simulink model "sst_dab_ttype_inv"  (R2026a)
settings: Solver=ode23tb  StopTime=simlength  FixedStep=tc  MaxStep=glb_time.tc
values from neighbouring files (symbols this model uses):
  afe_ctrl = ctrl_afe_setup(glb_time.ts_afe, grid_emu.omega_grid_nom)    [init_model.m]
  glb_time = timing_setup(fpwm_afe, trgo_afe, fpwm_inv, trgo_inv, fpwm_dab, trgo_dab,                  fpwm_cllc, trgo_cllc, t_measure, tc_factor, tc_decimation, delay_pwm, dead_time_afe,                  dead_time_inv, dead_time_dab, dead_time_cllc)    [init_model.m]
  grid_emu = grid_three_phase_emulator('Dyn11', delta_star, grid_nominal_power, application_voltage, us1, us2, fgrid,                  eq_grid_inductance, eq_grid_resistance, eta, ucc, i1m, p_iron, n1, n2, core_area, core_length, mur,                  up_xi_pu_ref, up_eta_pu_ref, un_xi_pu_ref, un_eta_pu_ref)    [init_model.m]
  omega_set = frequency_set*2*pi    (= 314.159265359)    [init_model.m]
  single_phase_inverter_ctrl = ctrl_single_phase_inverter_setup(glb_time.ts_inv, pres_ctrl.omega_set,      dqvector_pi.kp_inv, dqvector_pi.ki_inv, pres_ctrl.kp_rpi, pres_ctrl.ki_rpi, pres_ctrl.delta_rpi)    [init_model.m]
  sst_num_of_modules = 2    [init_model.m]
undefined symbols (not defined in the file or in its folder): hwdata
libraries: fl_lib x66, nesl_utility x38, pi_ctrl x4, full_bridge_ideal_switch x4, full_bridge_mosfet_based_with_thermal_model x4, full_bridge_mosfet_based_with_thermal_model_zvs x4, discrete_time_low_pass_filter x4, lithium_ion_battery x2, dab_single_phase_pwm_modulator x2, single_phase_transformer x2, dclink_for_three_levels x2, full_bridge_three_level_ttype_ideal_switch_based_model x2
(part 4 of 5)

== system sst_dab_ttype_inv/dab_modA/dcdc_with_galvanic_isolation/full-bridge_2/full-bridge_mosfet_based_with_thermal_model_zvs ==
  gate_commands : Inport
  data_measure : Subsystem
  full-bridge_mosfet_based_ with_thermal_model_zvs : full_bridge_mosfet_based_with_thermal_model_zvs/full-bridge_mosfet_based_ with_thermal_model_zvs  mass_heatsink_m=heatsink.no_weight  specific_heat_m=heatsink.cp  rth_mosfet_HA_m=heatsink.Rth_mosfet_HA  rth_mosfet_JH_m=mosfet.dab.Rth_mosfet_JH  Rds_on_m=mosfet.dab.Rds_on  Vth_m=mosfet.dab.Vth  Eon_m=mosfet.dab.Eon  Eoff_m=mosfet.dab.Eoff  Voff_sw_loss_m=mosfet.dab.Voff_sw_losses  Ion_sw_loss_m=mosfet.dab.Ion_sw_losses  Vdon_diode_m=mosfet.dab.Vdon_diode  Rdon_diode_m=mosfet.dab.Rds_on  JunctionTermalMass_m=mosfet.dab.JunctionTermalMass  Tambient_m=heatsink.Tambient  DThs_init_m=heatsink.DThs_init  Csnubber_m=mosfet.dab.Csnubber_zvs  Rsnubber_m=mosfet.dab.Rsnubber_zvs
  udc(+) : PMIOPort  Side=Left
  udc(-) : PMIOPort  Port=2  Side=Left
  uac(+) : PMIOPort  Port=3  Side=Right
  uac(-) : PMIOPort  Port=4  Side=Right
  wires:
  full-bridge_mosfet_based_ with_thermal_model_zvs/1 -> data_measure/1(m)
  gate_commands/1 -> full-bridge_mosfet_based_ with_thermal_model_zvs/1
  connections:
  full-bridge_mosfet_based_ with_thermal_model_zvs/LConn2 -- udc(-)/RConn1
  full-bridge_mosfet_based_ with_thermal_model_zvs/LConn1 -- udc(+)/RConn1
  full-bridge_mosfet_based_ with_thermal_model_zvs/RConn2 -- uac(-)/RConn1
  full-bridge_mosfet_based_ with_thermal_model_zvs/RConn1 -- uac(+)/RConn1

== system sst_dab_ttype_inv/dab_modB/dab_ctrl/dab_voltage&current_controllers/input current controller ==
  i_in_dab_ref : Inport
  i_in_dab : Inport  Port=2
  Gain : Gain
  dab_current_control performance_modA : Scope  NumInputPorts=3
      settings: ActiveDisplayYMinimum=-1.3198512407012277  ActiveDisplayYMaximum=3.2550260581251234  DataLoggingVariableName=ScopeData12
  pi_ctrl : pi_ctrl/pi_ctrl  kp=dab_ctrl.kp_idc  ki=dab_ctrl.ki_idc  ts=glb_time.ts_dab  lim_up=1  lim_down=-1
  i_ctrl_out : Outport
  wires:
  i_in_dab_ref/1 -> pi_ctrl/1, dab_current_control performance_modA/1, Gain/1  "i_in_dab_ref"
  i_in_dab/1 -> pi_ctrl/2, dab_current_control performance_modA/2  "i_in_dab"
  pi_ctrl/1 -> i_ctrl_out/1, dab_current_control performance_modA/3  "i_ctrl_out"
  Gain/1 -> pi_ctrl/3

== system sst_dab_ttype_inv/dab_modB/dab_ctrl/dab_voltage&current_controllers/output voltage controller ==
  u_out_dab_ref : Inport
  u_out_dab : Inport  Port=2
  dab_voltage_control performance_modA : Scope  NumInputPorts=3
      settings: ActiveDisplayYMinimum=-1.3198512407012277  ActiveDisplayYMaximum=3.2550260581251234  DataLoggingVariableName=ScopeData14
  pi_ctrl : pi_ctrl/pi_ctrl  kp=dab_ctrl.kp_udc  ki=dab_ctrl.ki_udc  ts=glb_time.ts_dab  lim_up=1  lim_down=-1
  u_ctrl_out : Outport
  wires:
  u_out_dab/1 -> dab_voltage_control performance_modA/2, pi_ctrl/2  "u_out_dab"
  u_out_dab_ref/1 -> dab_voltage_control performance_modA/1, pi_ctrl/3, pi_ctrl/1  "u_out_dab_ref"
  pi_ctrl/1 -> dab_voltage_control performance_modA/3, u_ctrl_out/1  "u_ctrl_out"

== system sst_dab_ttype_inv/dab_modB/dab_ctrl/dab_voltage&current_controllers/scopes ==
  Bus Creator : BusCreator  Inputs=2
  Bus Creator1 : BusCreator  Inputs=2
  dab-tracking modA : Scope  NumInputPorts=2
      settings: ActiveDisplayYMinimum=-2.2033655574404327  ActiveDisplayYMaximum=2.9011172646804795  DataLoggingVariableName=ScopeData7
  u_ctrl_out_dab/i_ctrl_out_dab modA : Scope  NumInputPorts=2
      settings: ActiveDisplayYMinimum=-1.25  ActiveDisplayYMaximum=1.25
  wires:
  [dab_current_input_pu] -> Bus Creator1/2  "dab_current_input_pu"
  [dab_current_ctrl_output_pu] -> u_ctrl_out_dab/i_ctrl_out_dab modA/2  "i_ctrl_out_dab"
  [dab_voltage_output_pu] -> Bus Creator/2  "dab_voltage_output_pu"
  [dab_voltage_output_pu_reference] -> Bus Creator/1  "dab_current_input_pu_ref"
  Bus Creator1/1 -> dab-tracking modA/2
  Bus Creator/1 -> dab-tracking modA/1
  [dab_voltage_ctrl_output_pu] -> u_ctrl_out_dab/i_ctrl_out_dab modA/1  "u_ctrl_out_dab"
  [dab_voltage_ctrl_output_pu] -> Bus Creator1/1  "u_ctrl_out_dab"

== system sst_dab_ttype_inv/dab_modB/dab_ctrl/dab_voltage&current_controllers/storage_data_dab ==
  To Workspace1 : ToWorkspace  VariableName=time_ts_dab_sim  SampleTime=-1
      settings: MaxDataPoints=Ns_dab
  To Workspace2 : ToWorkspace  VariableName=dab_current_input_pu_ref_sim  SampleTime=-1
      settings: MaxDataPoints=Ns_dab
  To Workspace3 : ToWorkspace  VariableName=dab_voltage_output_pu_sim  SampleTime=-1
      settings: MaxDataPoints=Ns_dab
  To Workspace5 : ToWorkspace  VariableName=dab_current_input_pu_sim  SampleTime=-1
      settings: MaxDataPoints=Ns_dab
  To Workspace6 : ToWorkspace  VariableName=u_ctrl_out_dab_sim  SampleTime=-1
      settings: MaxDataPoints=Ns_dab
  To Workspace7 : ToWorkspace  VariableName=i_ctrl_out_dab_sim  SampleTime=-1
      settings: MaxDataPoints=Ns_dab
  wires:
  [dab_voltage_ctrl_output_pu] -> To Workspace6/1  "u_ctrl_out_dab"
  [dab_voltage_output_pu_reference] -> To Workspace2/1  "dab_current_input_pu_ref"
  [dab_voltage_output_pu] -> To Workspace3/1  "dab_voltage_output_pu"
  [dab_current_ctrl_output_pu] -> To Workspace7/1  "i_ctrl_out_dab"
  [dab_current_input_pu] -> To Workspace5/1  "dab_current_input_pu"
  [time_dab_module_2] -> To Workspace1/1

== system sst_dab_ttype_inv/dab_modB/dcdc_with_galvanic_isolation/full-bridge_1/full-bridge_ideal_switch_based ==
  gate_commands : Inport
  data_measure : Subsystem
  full-bridge_ideal_switch_based : full_bridge_ideal_switch/full-bridge ideal switch based  Rds_on=ideal_switch.dab.Rds_on  Vdon_diode=ideal_switch.dab.Vdon_diode  Rdon_diode=ideal_switch.dab.Rdon_diode  Csnubber=ideal_switch.dab.Csnubber_zvs  Rsnubber=ideal_switch.dab.Rsnubber_zvs  Vth=ideal_switch.dab.Vth
  udc(+) : PMIOPort  Side=Left
  uac(+) : PMIOPort  Port=2  Side=Right
  udc(-) : PMIOPort  Port=3  Side=Left
  uac(-) : PMIOPort  Port=4  Side=Right
  wires:
  gate_commands/1 -> full-bridge_ideal_switch_based/1
  full-bridge_ideal_switch_based/1 -> data_measure/1(m)
  connections:
  uac(-)/RConn1 -- full-bridge_ideal_switch_based/RConn2
  full-bridge_ideal_switch_based/RConn1 -- uac(+)/RConn1
  udc(-)/RConn1 -- full-bridge_ideal_switch_based/LConn2
  udc(+)/RConn1 -- full-bridge_ideal_switch_based/LConn1

== system sst_dab_ttype_inv/dab_modB/dcdc_with_galvanic_isolation/full-bridge_1/full-bridge_mosfet_based_with_thermal_model ==
  gate_commands : Inport
  data_measure : Subsystem
  full-bridge_mosfet_based_with_thermal_model : full_bridge_mosfet_based_with_thermal_model/full-bridge mosfet based with thermal model  mass_heatsink_m=heatsink.no_weight  specific_heat_m=heatsink.cp  rth_mosfet_HA_m=heatsink.Rth_mosfet_HA  rth_mosfet_JH_m=mosfet.dab.Rth_mosfet_JH  Rds_on_m=mosfet.dab.Rds_on  Vth_m=mosfet.dab.Vth  Eon_m=mosfet.dab.Eon  Eoff_m=mosfet.dab.Eoff  Voff_sw_loss_m=mosfet.dab.Voff_sw_losses  Ion_sw_loss_m=mosfet.dab.Ion_sw_losses  Vdon_diode_m=mosfet.dab.Vdon_diode  Rdon_diode_m=mosfet.dab.Rds_on  JunctionTermalMass_m=mosfet.dab.JunctionTermalMass  Tambient_m=heatsink.Tambient  DThs_init_m=heatsink.DThs_init
  udc(+) : PMIOPort  Side=Left
  uac(+) : PMIOPort  Port=2  Side=Right
  udc(-) : PMIOPort  Port=3  Side=Left
  uac(-) : PMIOPort  Port=4  Side=Right
  wires:
  gate_commands/1 -> full-bridge_mosfet_based_with_thermal_model/1
  full-bridge_mosfet_based_with_thermal_model/1 -> data_measure/1(m)
  connections:
  full-bridge_mosfet_based_with_thermal_model/RConn1 -- uac(+)/RConn1
  udc(-)/RConn1 -- full-bridge_mosfet_based_with_thermal_model/LConn2
  full-bridge_mosfet_based_with_thermal_model/LConn1 -- udc(+)/RConn1
  full-bridge_mosfet_based_with_thermal_model/RConn2 -- uac(-)/RConn1

== system sst_dab_ttype_inv/dab_modB/dcdc_with_galvanic_isolation/full-bridge_1/full-bridge_mosfet_based_with_thermal_model_zvs ==
  gate_commands : Inport
  data_measure : Subsystem
  full-bridge_mosfet_based_ with_thermal_model_zvs : full_bridge_mosfet_based_with_thermal_model_zvs/full-bridge_mosfet_based_ with_thermal_model_zvs  mass_heatsink_m=heatsink.no_weight  specific_heat_m=heatsink.cp  rth_mosfet_HA_m=heatsink.Rth_mosfet_HA  rth_mosfet_JH_m=mosfet.dab.Rth_mosfet_JH  Rds_on_m=mosfet.dab.Rds_on  Vth_m=mosfet.dab.Vth  Eon_m=mosfet.dab.Eon  Eoff_m=mosfet.dab.Eoff  Voff_sw_loss_m=mosfet.dab.Voff_sw_losses  Ion_sw_loss_m=mosfet.dab.Ion_sw_losses  Vdon_diode_m=mosfet.dab.Vdon_diode  Rdon_diode_m=mosfet.dab.Rds_on  JunctionTermalMass_m=mosfet.dab.JunctionTermalMass  Tambient_m=heatsink.Tambient  DThs_init_m=heatsink.DThs_init  Csnubber_m=mosfet.dab.Csnubber_zvs  Rsnubber_m=mosfet.dab.Rsnubber_zvs
  udc(+) : PMIOPort  Side=Left
  udc(-) : PMIOPort  Port=2  Side=Left
  uac(+) : PMIOPort  Port=3  Side=Right
  uac(-) : PMIOPort  Port=4  Side=Right
  wires:
  gate_commands/1 -> full-bridge_mosfet_based_ with_thermal_model_zvs/1
  full-bridge_mosfet_based_ with_thermal_model_zvs/1 -> data_measure/1(m)
  connections:
  full-bridge_mosfet_based_ with_thermal_model_zvs/RConn1 -- uac(+)/RConn1
  full-bridge_mosfet_based_ with_thermal_model_zvs/RConn2 -- uac(-)/RConn1
  full-bridge_mosfet_based_ with_thermal_model_zvs/LConn1 -- udc(+)/RConn1
  full-bridge_mosfet_based_ with_thermal_model_zvs/LConn2 -- udc(-)/RConn1

== system sst_dab_ttype_inv/dab_modB/dcdc_with_galvanic_isolation/full-bridge_2/full-bridge_ideal_switch_based ==
  gate_commands : Inport
  data_measure : Subsystem
  full-bridge_ideal_switch_based : full_bridge_ideal_switch/full-bridge ideal switch based  Rds_on=ideal_switch.dab.Rds_on  Vdon_diode=ideal_switch.dab.Vdon_diode  Rdon_diode=ideal_switch.dab.Rdon_diode  Csnubber=ideal_switch.dab.Csnubber_zvs  Rsnubber=ideal_switch.dab.Rsnubber_zvs  Vth=ideal_switch.dab.Vth
  udc(+) : PMIOPort  Side=Left
  uac(+) : PMIOPort  Port=2  Side=Right
  udc(-) : PMIOPort  Port=3  Side=Left
  uac(-) : PMIOPort  Port=4  Side=Right
  wires:
  gate_commands/1 -> full-bridge_ideal_switch_based/1
  full-bridge_ideal_switch_based/1 -> data_measure/1(m)
  connections:
  uac(-)/RConn1 -- full-bridge_ideal_switch_based/RConn2
  full-bridge_ideal_switch_based/RConn1 -- uac(+)/RConn1
  udc(-)/RConn1 -- full-bridge_ideal_switch_based/LConn2
  udc(+)/RConn1 -- full-bridge_ideal_switch_based/LConn1

== system sst_dab_ttype_inv/dab_modB/dcdc_with_galvanic_isolation/full-bridge_2/full-bridge_mosfet_based_with_thermal_model ==
  gate_commands : Inport
  data_measure : Subsystem
  full-bridge_mosfet_based_with_thermal_model : full_bridge_mosfet_based_with_thermal_model/full-bridge mosfet based with thermal model  mass_heatsink_m=heatsink.no_weight  specific_heat_m=heatsink.cp  rth_mosfet_HA_m=heatsink.Rth_mosfet_HA  rth_mosfet_JH_m=mosfet.dab.Rth_mosfet_JH  Rds_on_m=mosfet.dab.Rds_on  Vth_m=mosfet.dab.Vth  Eon_m=mosfet.dab.Eon  Eoff_m=mosfet.dab.Eoff  Voff_sw_loss_m=mosfet.dab.Voff_sw_losses  Ion_sw_loss_m=mosfet.dab.Ion_sw_losses  Vdon_diode_m=mosfet.dab.Vdon_diode  Rdon_diode_m=mosfet.dab.Rds_on  JunctionTermalMass_m=mosfet.dab.JunctionTermalMass  Tambient_m=heatsink.Tambient  DThs_init_m=heatsink.DThs_init
  udc(+) : PMIOPort  Side=Left
  uac(+) : PMIOPort  Port=2  Side=Right
  udc(-) : PMIOPort  Port=3  Side=Left
  uac(-) : PMIOPort  Port=4  Side=Right
  wires:
  gate_commands/1 -> full-bridge_mosfet_based_with_thermal_model/1
  full-bridge_mosfet_based_with_thermal_model/1 -> data_measure/1(m)
  connections:
  full-bridge_mosfet_based_with_thermal_model/RConn1 -- uac(+)/RConn1
  udc(-)/RConn1 -- full-bridge_mosfet_based_with_thermal_model/LConn2
  full-bridge_mosfet_based_with_thermal_model/LConn1 -- udc(+)/RConn1
  full-bridge_mosfet_based_with_thermal_model/RConn2 -- uac(-)/RConn1

== system sst_dab_ttype_inv/dab_modB/dcdc_with_galvanic_isolation/full-bridge_2/full-bridge_mosfet_based_with_thermal_model_zvs ==
  gate_commands : Inport
  data_measure : Subsystem
  full-bridge_mosfet_based_ with_thermal_model_zvs : full_bridge_mosfet_based_with_thermal_model_zvs/full-bridge_mosfet_based_ with_thermal_model_zvs  mass_heatsink_m=heatsink.no_weight  specific_heat_m=heatsink.cp  rth_mosfet_HA_m=heatsink.Rth_mosfet_HA  rth_mosfet_JH_m=mosfet.dab.Rth_mosfet_JH  Rds_on_m=mosfet.dab.Rds_on  Vth_m=mosfet.dab.Vth  Eon_m=mosfet.dab.Eon  Eoff_m=mosfet.dab.Eoff  Voff_sw_loss_m=mosfet.dab.Voff_sw_losses  Ion_sw_loss_m=mosfet.dab.Ion_sw_losses  Vdon_diode_m=mosfet.dab.Vdon_diode  Rdon_diode_m=mosfet.dab.Rds_on  JunctionTermalMass_m=mosfet.dab.JunctionTermalMass  Tambient_m=heatsink.Tambient  DThs_init_m=heatsink.DThs_init  Csnubber_m=mosfet.dab.Csnubber_zvs  Rsnubber_m=mosfet.dab.Rsnubber_zvs
  udc(+) : PMIOPort  Side=Left
  udc(-) : PMIOPort  Port=2  Side=Left
  uac(+) : PMIOPort  Port=3  Side=Right
  uac(-) : PMIOPort  Port=4  Side=Right
  wires:
  gate_commands/1 -> full-bridge_mosfet_based_ with_thermal_model_zvs/1
  full-bridge_mosfet_based_ with_thermal_model_zvs/1 -> data_measure/1(m)
  connections:
  full-bridge_mosfet_based_ with_thermal_model_zvs/RConn1 -- uac(+)/RConn1
  full-bridge_mosfet_based_ with_thermal_model_zvs/RConn2 -- uac(-)/RConn1
  full-bridge_mosfet_based_ with_thermal_model_zvs/LConn1 -- udc(+)/RConn1
  full-bridge_mosfet_based_ with_thermal_model_zvs/LConn2 -- udc(-)/RConn1

== system sst_dab_ttype_inv/single_phase_inverter_modA/single phase inverter control/single_phase_inverter_ctrl/scopes ==
  Bus Creator1 : BusCreator  Inputs=3
  Bus Creator2 : BusCreator  Inputs=2
  Bus Creator3 : BusCreator  Inputs=2
  Bus Creator4 : BusCreator  Inputs=2
  single phase inverter tracking current scope 1 : Scope  NumInputPorts=2
      settings: ActiveDisplayYMinimum=-1.23468017578125  ActiveDisplayYMaximum=1.23419189453125  DataLoggingVariableName=ScopeData12
  single phase inverter tracking current scope 2 : Scope  NumInputPorts=2
      settings: ActiveDisplayYMinimum=-3.07452392578125  ActiveDisplayYMaximum=2.19708251953125  DataLoggingVariableName=ScopeData2
  wires:
  Bus Creator1/1 -> single phase inverter tracking current scope 1/2  "is_tracking"
  [i_out_alphabeta_ref] -> Bus Creator1/2  "i_out_inverter_pu_ref"
  [afe_current_output_pu] -> Bus Creator1/3  "inverter_current_output_pu"
  [afe_voltage_output_pu] -> Bus Creator2/1  "inverter_voltage_output_pu"
  Bus Creator2/1 -> single phase inverter tracking current scope 1/1  "load"
  [inverter_current_output_pu_reference] -> Bus Creator1/1  "inverter_current_output_pu_reference"
  [afe_current_output_pu] -> Bus Creator2/2  "inverter_current_output_pu"
  [u_ctrl_out] -> Bus Creator3/1  "u_ctrl_out"
  [afe_voltage_output_pu] -> Bus Creator3/2  "inverter_voltage_output_pu"
  Bus Creator3/1 -> single phase inverter tracking current scope 2/2  "u_load"
  [afe_current_output_pu] -> Bus Creator4/2  "inverter_current_output_pu"
  [i_out_alphabeta_ref] -> Bus Creator4/1  "i_out_alphabeta_ref"
  Bus Creator4/1 -> single phase inverter tracking current scope 2/1  "i_load"

== system sst_dab_ttype_inv/single_phase_inverter_modA/single phase inverter control/single_phase_inverter_ctrl/single_phase_current_control ==
  inverter_current_output_pu_reference : Inport
  current_reference_generation : Subsystem
  dqpi_current_controller : Subsystem
  u_ctrl_out : Outport
  tag scope: i_out_alphabeta_ref=scoped, inverter_current_output_pu_reference=scoped, u_ctrl_out=scoped
  wires:
  current_reference_generation/1(is_ref) -> [i_out_alphabeta_ref]  "i_out_inverter_pu_ref"
  dqpi_current_controller/1(u_out) -> u_ctrl_out/1, [u_ctrl_out]  "u_ctrl_out"
  [phase_grid] -> current_reference_generation/2(phase)
  inverter_current_output_pu_reference/1 -> current_reference_generation/1(mag_ref), [inverter_current_output_pu_reference]
  current_reference_generation/2(id_ref) -> dqpi_current_controller/1(id_ref)

== system sst_dab_ttype_inv/single_phase_inverter_modA/single phase inverter control/single_phase_inverter_ctrl/single_phase_pll ==
  input : Inport
  Constant : Constant
  Constant2 : Constant  Value=0
  Scope : Scope  NumInputPorts=2
      settings: ActiveDisplayYMinimum=-3.2854912154015015  ActiveDisplayYMaximum=3.4773424919151528
  Sum : Sum  Inputs=|++
  Sum1 : Sum  Inputs=|++
  Terminator : Terminator
  Terminator1 : Terminator
  Terminator2 : Terminator
  Unit Delay1 : UnitDelay  SampleTime=-1
  alphabeta2xieta : MATLAB Function  TreatAsAtomicUnit=on
  bounder2 : MATLAB Function  TreatAsAtomicUnit=on
  double_integrator_observer : Subsystem
  freq_pll : Gain  Gain=1/2/pi
  omega_int_ts : Gain  Gain=omega_set * glb_time.ts_inv
  pi-ctrl : Subsystem  mask{kp=1, ki=0, ts=glb_time.ts_inv, sat_pos=2, sat_neg=-2}
  ualpha_pll : Gain
  ubeta_pll : Gain
  ueta_pll : Gain  Gain=-1
  ueta_pll_flt : discrete_time_low_pass_filter/discrete-time-low-pass-filter  tau=2/omega_set  ts=glb_time.ts_inv
  uxi_pll : Gain
  uxi_pll_flt : discrete_time_low_pass_filter/discrete-time-low-pass-filter  tau=2/omega_set  ts=glb_time.ts_inv
  xieta2alphabeta : MATLAB Function  TreatAsAtomicUnit=on
  phase_pll_hat : Outport
  omega_pll_hat : Outport  Port=2
  wires:
  Sum/1 -> bounder2/1(u)
  alphabeta2xieta/1(xi) -> uxi_pll/1, uxi_pll_flt/1
  xieta2alphabeta/2(beta) -> ubeta_pll/1
  alphabeta2xieta/2(eta) -> ueta_pll/1, ueta_pll_flt/1
  omega_int_ts/1 -> freq_pll/1, Sum/1
  double_integrator_observer/1(phase_hat) -> Scope/1, phase_pll_hat/1  "phase_pll_hat"
  input/1 -> alphabeta2xieta/1(alpha)
  freq_pll/1 -> Terminator1/1  "freq_pll"
  ueta_pll_flt/1 -> xieta2alphabeta/2(eta)
  uxi_pll_flt/1 -> xieta2alphabeta/1(xi)
  ueta_pll/1 -> pi-ctrl/1(x)
  Sum1/1 -> omega_int_ts/1  "freq_pll"
  Constant2/1 -> pi-ctrl/2(xref)
  uxi_pll/1 -> Terminator2/1
  ubeta_pll/1 -> alphabeta2xieta/2(beta)
  xieta2alphabeta/1(alpha) -> ualpha_pll/1
  pi-ctrl/1(u) -> Sum1/1
  Constant/1 -> Sum1/2
  Unit Delay1/1 -> Sum/2, alphabeta2xieta/3(gamma), xieta2alphabeta/3(gamma), double_integrator_observer/1(theta)
  bounder2/1(y) -> Unit Delay1/1  "theta_hat_bounded"
  double_integrator_observer/2(omega_hat) -> Scope/2, omega_pll_hat/1  "omega_pll_hat"
  ualpha_pll/1 -> Terminator/1

== system sst_dab_ttype_inv/single_phase_inverter_modA/single phase inverter control/single_phase_inverter_ctrl/storage_data ==
  To Workspace : ToWorkspace  VariableName=inverter_voltage_output_pu_sim  SampleTime=-1
      settings: MaxDataPoints=glb_time.Ns_inv  Save2DSignal=2-D array (concatenate along first dimension)
  To Workspace1 : ToWorkspace  VariableName=inverter_current_output_pu_sim  SampleTime=-1
      settings: MaxDataPoints=glb_time.Ns_inv  Save2DSignal=2-D array (concatenate along first dimension)
  To Workspace10 : ToWorkspace  VariableName=iq_pu_ref_sim  SampleTime=-1
      settings: MaxDataPoints=glb_time.Ns_inv  Save2DSignal=2-D array (concatenate along first dimension)
  To Workspace11 : ToWorkspace  VariableName=iq_pu_sim  SampleTime=-1
      settings: MaxDataPoints=glb_time.Ns_inv  Save2DSignal=2-D array (concatenate along first dimension)
  To Workspace12 : ToWorkspace  VariableName=ud_ctrl_out_sim  SampleTime=-1
      settings: MaxDataPoints=glb_time.Ns_inv  Save2DSignal=2-D array (concatenate along first dimension)
  To Workspace13 : ToWorkspace  VariableName=uq_ctrl_out_sim  SampleTime=-1
      settings: MaxDataPoints=glb_time.Ns_inv  Save2DSignal=2-D array (concatenate along first dimension)
  To Workspace2 : ToWorkspace  VariableName=inverter_current_output_pu_reference_sim  SampleTime=-1
      settings: MaxDataPoints=glb_time.Ns_inv  Save2DSignal=2-D array (concatenate along first dimension)
  To Workspace3 : ToWorkspace  VariableName=i_out_inverter_pu_ref_sim  SampleTime=-1
      settings: MaxDataPoints=glb_time.Ns_inv  Save2DSignal=2-D array (concatenate along first dimension)
  To Workspace4 : ToWorkspace  VariableName=u_ctrl_out_sim  SampleTime=-1
      settings: MaxDataPoints=glb_time.Ns_inv  Save2DSignal=2-D array (concatenate along first dimension)
  To Workspace5 : ToWorkspace  VariableName=time_ts_inv_sim  SampleTime=-1
      settings: MaxDataPoints=glb_time.Ns_inv  Save2DSignal=2-D array (concatenate along first dimension)
  To Workspace6 : ToWorkspace  VariableName=i_alpha_pu_sim  SampleTime=-1
      settings: MaxDataPoints=glb_time.Ns_inv  Save2DSignal=2-D array (concatenate along first dimension)
  To Workspace7 : ToWorkspace  VariableName=i_beta_pu_sim  SampleTime=-1
      settings: MaxDataPoints=glb_time.Ns_inv  Save2DSignal=2-D array (concatenate along first dimension)
  To Workspace8 : ToWorkspace  VariableName=id_pu_ref_sim  SampleTime=-1
      settings: MaxDataPoints=glb_time.Ns_inv  Save2DSignal=2-D array (concatenate along first dimension)
  To Workspace9 : ToWorkspace  VariableName=id_pu_sim  SampleTime=-1
      settings: MaxDataPoints=glb_time.Ns_inv  Save2DSignal=2-D array (concatenate along first dimension)
  wires:
  [afe_voltage_output_pu] -> To Workspace/1  "inverter_voltage_output_pu"
  [afe_current_output_pu] -> To Workspace1/1  "inverter_current_output_pu"
  [inverter_current_output_pu_reference] -> To Workspace2/1  "inverter_current_output_pu_reference"
  [i_out_alphabeta_ref] -> To Workspace3/1  "i_out_inverter_pu_ref"
  [u_ctrl_out] -> To Workspace4/1  "u_ctrl_out"
  [local_time] -> To Workspace5/1
  [i_alpha] -> To Workspace6/1
  [i_beta] -> To Workspace7/1
  [id_ref] -> To Workspace8/1
  [id] -> To Workspace9/1
  [iq_ref] -> To Workspace10/1
  [iq] -> To Workspace11/1
  [ud_ctrl] -> To Workspace12/1
  [uq_ctrl] -> To Workspace13/1

== system sst_dab_ttype_inv/single_phase_inverter_modB/single phase inverter control/single_phase_inverter_ctrl/scopes ==
  Bus Creator1 : BusCreator  Inputs=3
  Bus Creator2 : BusCreator  Inputs=2
  Bus Creator3 : BusCreator  Inputs=2
  Bus Creator4 : BusCreator  Inputs=2
  single phase inverter tracking current scope 1 : Scope  NumInputPorts=2
      settings: ActiveDisplayYMinimum=-1.23468017578125  ActiveDisplayYMaximum=1.23419189453125  DataLoggingVariableName=ScopeData12
  single phase inverter tracking current scope 2 : Scope  NumInputPorts=2
      settings: ActiveDisplayYMinimum=-1.2603759765625  ActiveDisplayYMaximum=1.2652587890625  DataLoggingVariableName=ScopeData2
  wires:
  Bus Creator4/1 -> single phase inverter tracking current scope 2/1  "i_load"
  [i_out_alphabeta_ref] -> Bus Creator4/1  "i_out_alphabeta_ref"
  [afe_current_output_pu] -> Bus Creator4/2  "inverter_current_output_pu"
  Bus Creator3/1 -> single phase inverter tracking current scope 2/2  "u_load"
  [afe_voltage_output_pu] -> Bus Creator3/2  "inverter_voltage_output_pu"
  [u_ctrl_out] -> Bus Creator3/1  "u_ctrl_out"
  [afe_current_output_pu] -> Bus Creator2/2  "inverter_current_output_pu"
  [inverter_current_output_pu_reference] -> Bus Creator1/1  "inverter_current_output_pu_reference"
  Bus Creator2/1 -> single phase inverter tracking current scope 1/1  "load"
  [afe_voltage_output_pu] -> Bus Creator2/1  "inverter_voltage_output_pu"
  [afe_current_output_pu] -> Bus Creator1/3  "inverter_current_output_pu"
  [i_out_alphabeta_ref] -> Bus Creator1/2  "i_out_inverter_pu_ref"
  Bus Creator1/1 -> single phase inverter tracking current scope 1/2  "is_tracking"

== system sst_dab_ttype_inv/single_phase_inverter_modB/single phase inverter control/single_phase_inverter_ctrl/single_phase_current_control ==
  inverter_current_output_pu_reference : Inport
  current_reference_generation : Subsystem
  dqpi_current_controller : Subsystem
  u_ctrl_out : Outport
  tag scope: i_out_alphabeta_ref=scoped, inverter_current_output_pu_reference=scoped, u_ctrl_out=scoped
  wires:
  current_reference_generation/2(id_ref) -> dqpi_current_controller/1(id_ref)
  inverter_current_output_pu_reference/1 -> [inverter_current_output_pu_reference], current_reference_generation/1(mag_ref)
  [phase_grid] -> current_reference_generation/2(phase)
  dqpi_current_controller/1(u_out) -> [u_ctrl_out], u_ctrl_out/1  "u_ctrl_out"
  current_reference_generation/1(is_ref) -> [i_out_alphabeta_ref]  "i_out_inverter_pu_ref"

== system sst_dab_ttype_inv/single_phase_inverter_modB/single phase inverter control/single_phase_inverter_ctrl/single_phase_pll ==
  input : Inport
  Constant : Constant
  Constant2 : Constant  Value=0
  Scope : Scope  NumInputPorts=2
      settings: ActiveDisplayYMinimum=-3.2854912154015015  ActiveDisplayYMaximum=3.4773424919151528
  Sum : Sum  Inputs=|++
  Sum1 : Sum  Inputs=|++
  Terminator : Terminator
  Terminator1 : Terminator
  Terminator2 : Terminator
  Unit Delay1 : UnitDelay  SampleTime=-1
  alphabeta2xieta : MATLAB Function  TreatAsAtomicUnit=on
  bounder2 : MATLAB Function  TreatAsAtomicUnit=on
  double_integrator_observer : Subsystem
  freq_pll : Gain  Gain=1/2/pi
  omega_int_ts : Gain  Gain=omega_set * glb_time.ts_inv
  pi-ctrl : Subsystem  mask{kp=1, ki=0, ts=glb_time.ts_inv, sat_pos=2, sat_neg=-2}
  ualpha_pll : Gain
  ubeta_pll : Gain
  ueta_pll : Gain  Gain=-1
  ueta_pll_flt : discrete_time_low_pass_filter/discrete-time-low-pass-filter  tau=2/omega_set  ts=glb_time.ts_inv
  uxi_pll : Gain
  uxi_pll_flt : discrete_time_low_pass_filter/discrete-time-low-pass-filter  tau=2/omega_set  ts=glb_time.ts_inv
  xieta2alphabeta : MATLAB Function  TreatAsAtomicUnit=on
  phase_pll_hat : Outport
  omega_pll_hat : Outport  Port=2
  wires:
  ualpha_pll/1 -> Terminator/1
  double_integrator_observer/2(omega_hat) -> omega_pll_hat/1, Scope/2  "omega_pll_hat"
  bounder2/1(y) -> Unit Delay1/1  "theta_hat_bounded"
  Unit Delay1/1 -> double_integrator_observer/1(theta), xieta2alphabeta/3(gamma), alphabeta2xieta/3(gamma), Sum/2
  Constant/1 -> Sum1/2
  pi-ctrl/1(u) -> Sum1/1
  xieta2alphabeta/1(alpha) -> ualpha_pll/1
  ubeta_pll/1 -> alphabeta2xieta/2(beta)
  uxi_pll/1 -> Terminator2/1
  Constant2/1 -> pi-ctrl/2(xref)
  Sum1/1 -> omega_int_ts/1  "freq_pll"
  ueta_pll/1 -> pi-ctrl/1(x)
  uxi_pll_flt/1 -> xieta2alphabeta/1(xi)
  ueta_pll_flt/1 -> xieta2alphabeta/2(eta)
  freq_pll/1 -> Terminator1/1  "freq_pll"
  input/1 -> alphabeta2xieta/1(alpha)
  double_integrator_observer/1(phase_hat) -> phase_pll_hat/1, Scope/1  "phase_pll_hat"
  omega_int_ts/1 -> Sum/1, freq_pll/1
  alphabeta2xieta/2(eta) -> ueta_pll_flt/1, ueta_pll/1
  xieta2alphabeta/2(beta) -> ubeta_pll/1
  alphabeta2xieta/1(xi) -> uxi_pll_flt/1, uxi_pll/1
  Sum/1 -> bounder2/1(u)

== system sst_dab_ttype_inv/single_phase_inverter_modB/single phase inverter control/single_phase_inverter_ctrl/storage_data ==
  To Workspace : ToWorkspace  VariableName=inverter_voltage_output_pu_sim  SampleTime=-1
      settings: MaxDataPoints=glb_time.Ns_inv  Save2DSignal=2-D array (concatenate along first dimension)
  To Workspace1 : ToWorkspace  VariableName=inverter_current_output_pu_sim  SampleTime=-1
      settings: MaxDataPoints=glb_time.Ns_inv  Save2DSignal=2-D array (concatenate along first dimension)
  To Workspace10 : ToWorkspace  VariableName=iq_pu_ref_sim  SampleTime=-1
      settings: MaxDataPoints=glb_time.Ns_inv  Save2DSignal=2-D array (concatenate along first dimension)
  To Workspace11 : ToWorkspace  VariableName=iq_pu_sim  SampleTime=-1
      settings: MaxDataPoints=glb_time.Ns_inv  Save2DSignal=2-D array (concatenate along first dimension)
  To Workspace12 : ToWorkspace  VariableName=ud_ctrl_out_sim  SampleTime=-1
      settings: MaxDataPoints=glb_time.Ns_inv  Save2DSignal=2-D array (concatenate along first dimension)
  To Workspace13 : ToWorkspace  VariableName=uq_ctrl_out_sim  SampleTime=-1
      settings: MaxDataPoints=glb_time.Ns_inv  Save2DSignal=2-D array (concatenate along first dimension)
  To Workspace2 : ToWorkspace  VariableName=inverter_current_output_pu_reference_sim  SampleTime=-1
      settings: MaxDataPoints=glb_time.Ns_inv  Save2DSignal=2-D array (concatenate along first dimension)
  To Workspace3 : ToWorkspace  VariableName=i_out_inverter_pu_ref_sim  SampleTime=-1
      settings: MaxDataPoints=glb_time.Ns_inv  Save2DSignal=2-D array (concatenate along first dimension)
  To Workspace4 : ToWorkspace  VariableName=u_ctrl_out_sim  SampleTime=-1
      settings: MaxDataPoints=glb_time.Ns_inv  Save2DSignal=2-D array (concatenate along first dimension)
  To Workspace5 : ToWorkspace  VariableName=time_ts_inv_sim  SampleTime=-1
      settings: MaxDataPoints=glb_time.Ns_inv  Save2DSignal=2-D array (concatenate along first dimension)
  To Workspace6 : ToWorkspace  VariableName=i_alpha_pu_sim  SampleTime=-1
      settings: MaxDataPoints=glb_time.Ns_inv  Save2DSignal=2-D array (concatenate along first dimension)
  To Workspace7 : ToWorkspace  VariableName=i_beta_pu_sim  SampleTime=-1
      settings: MaxDataPoints=glb_time.Ns_inv  Save2DSignal=2-D array (concatenate along first dimension)
  To Workspace8 : ToWorkspace  VariableName=id_pu_ref_sim  SampleTime=-1
      settings: MaxDataPoints=glb_time.Ns_inv  Save2DSignal=2-D array (concatenate along first dimension)
  To Workspace9 : ToWorkspace  VariableName=id_pu_sim  SampleTime=-1
      settings: MaxDataPoints=glb_time.Ns_inv  Save2DSignal=2-D array (concatenate along first dimension)
  wires:
  [uq_ctrl] -> To Workspace13/1
  [ud_ctrl] -> To Workspace12/1
  [iq] -> To Workspace11/1
  [iq_ref] -> To Workspace10/1
  [id] -> To Workspace9/1
  [id_ref] -> To Workspace8/1
  [i_beta] -> To Workspace7/1
  [i_alpha] -> To Workspace6/1
  [local_time] -> To Workspace5/1
  [u_ctrl_out] -> To Workspace4/1  "u_ctrl_out"
  [i_out_alphabeta_ref] -> To Workspace3/1  "i_out_inverter_pu_ref"
  [inverter_current_output_pu_reference] -> To Workspace2/1  "inverter_current_output_pu_reference"
  [afe_current_output_pu] -> To Workspace1/1  "inverter_current_output_pu"
  [afe_voltage_output_pu] -> To Workspace/1  "inverter_voltage_output_pu"

== system sst_dab_ttype_inv/dab_modA/dcdc_with_galvanic_isolation/full-bridge_1/full-bridge_ideal_switch_based/data_measure ==
  m : Inport
  Bus Selector1 : BusSelector  OutputSignals=ideal_switch_current_Q2,ideal_switch_voltage_Q2
  Bus Selector2 : BusSelector  OutputSignals=ideal_switch_current_Q1,ideal_switch_voltage_Q1
  tag scope: idevice_ids_dab_Q1_modA=global, idevice_ids_dab_Q2_modA=global, idevice_uds_dab_Q1_modA=global, idevice_uds_dab_Q2_modA=global
  wires:
  Bus Selector1/1 -> [idevice_ids_dab_Q2_modA]  "<ideal_switch_current_Q2>"
  Bus Selector1/2 -> [idevice_uds_dab_Q2_modA]  "<ideal_switch_voltage_Q2>"
  m/1 -> Bus Selector2/1, Bus Selector1/1
  Bus Selector2/1 -> [idevice_ids_dab_Q1_modA]  "<ideal_switch_current_Q1>"
  Bus Selector2/2 -> [idevice_uds_dab_Q1_modA]  "<ideal_switch_voltage_Q1>"

== system sst_dab_ttype_inv/dab_modA/dcdc_with_galvanic_isolation/full-bridge_1/full-bridge_mosfet_based_with_thermal_model/data_measure ==
  m : Inport
  Bus Selector : BusSelector  OutputSignals=mosfet_ploss_Q1,mosfet_voltage_Q1,mosfet_current_Q1,mosfet_JH_temp_Q1,mosfet_HA_temp_Q1
  Bus Selector1 : BusSelector  OutputSignals=mosfet_ploss_Q2,mosfet_voltage_Q2,mosfet_current_Q2,mosfet_JH_temp_Q2,mosfet_HA_temp_Q2
  tag scope: inverter_1_dab_mosfet_modA=global, mosfet_HA_temp_dab_Q1=global, mosfet_HA_temp_dab_Q2=global, mosfet_JH_temp_dab_Q1=global, mosfet_JH_temp_dab_Q2=global, mosfet_ids_dab_Q1=global, mosfet_ids_dab_Q2=global, mosfet_plosses_dab_Q1=global, mosfet_plosses_dab_Q2=global, mosfet_uds_dab_Q1=global, mosfet_uds_dab_Q2=global
  wires:
  Bus Selector/1 -> [mosfet_plosses_dab_Q1]  "<mosfet_ploss_Q1>"
  Bus Selector1/3 -> [mosfet_ids_dab_Q2]  "<mosfet_current_Q2>"
  Bus Selector1/2 -> [mosfet_uds_dab_Q2]  "<mosfet_voltage_Q2>"
  Bus Selector1/5 -> [mosfet_HA_temp_dab_Q2]  "<mosfet_HA_temp_Q2>"
  Bus Selector/4 -> [mosfet_JH_temp_dab_Q1]  "<mosfet_JH_temp_Q1>"
  Bus Selector/5 -> [mosfet_HA_temp_dab_Q1]  "<mosfet_HA_temp_Q1>"
  Bus Selector1/4 -> [mosfet_JH_temp_dab_Q2]  "<mosfet_JH_temp_Q2>"
  Bus Selector/3 -> [mosfet_ids_dab_Q1]  "<mosfet_current_Q1>"
  Bus Selector/2 -> [mosfet_uds_dab_Q1]  "<mosfet_voltage_Q1>"
  Bus Selector1/1 -> [mosfet_plosses_dab_Q2]  "<mosfet_ploss_Q2>"
  m/1 -> Bus Selector/1, Bus Selector1/1, [inverter_1_dab_mosfet_modA]

== system sst_dab_ttype_inv/dab_modA/dcdc_with_galvanic_isolation/full-bridge_1/full-bridge_mosfet_based_with_thermal_model_zvs/data_measure ==
  m : Inport
  Bus Selector : BusSelector  OutputSignals=mosfet_ploss_Q1,mosfet_voltage_Q1,mosfet_current_Q1,mosfet_JH_temp_Q1,mosfet_HA_temp_Q1
  Bus Selector1 : BusSelector  OutputSignals=mosfet_ploss_Q2,mosfet_voltage_Q2,mosfet_current_Q2,mosfet_JH_temp_Q2,mosfet_HA_temp_Q2
  tag scope: inverter_1_dab_mosfet_zvs_modA=global, mosfet_dab_HA_temp_dab_Q1=global, mosfet_dab_HA_temp_dab_Q2=global, mosfet_dab_JH_temp_dab_Q1=global, mosfet_dab_JH_temp_dab_Q2=global, mosfet_dab_ids_dab_Q1=global, mosfet_dab_ids_dab_Q2=global, mosfet_dab_plosses_dab_Q1=global, mosfet_dab_plosses_dab_Q2=global, mosfet_dab_uds_dab_Q1=global, mosfet_dab_uds_dab_Q2=global
  wires:
  Bus Selector/1 -> [mosfet_dab_plosses_dab_Q1]  "<mosfet_ploss_Q1>"
  Bus Selector1/3 -> [mosfet_dab_ids_dab_Q2]  "<mosfet_current_Q2>"
  Bus Selector1/2 -> [mosfet_dab_uds_dab_Q2]  "<mosfet_voltage_Q2>"
  Bus Selector1/5 -> [mosfet_dab_HA_temp_dab_Q2]  "<mosfet_HA_temp_Q2>"
  Bus Selector/4 -> [mosfet_dab_JH_temp_dab_Q1]  "<mosfet_JH_temp_Q1>"
  Bus Selector/5 -> [mosfet_dab_HA_temp_dab_Q1]  "<mosfet_HA_temp_Q1>"
  Bus Selector1/4 -> [mosfet_dab_JH_temp_dab_Q2]  "<mosfet_JH_temp_Q2>"
  Bus Selector/3 -> [mosfet_dab_ids_dab_Q1]  "<mosfet_current_Q1>"
  Bus Selector/2 -> [mosfet_dab_uds_dab_Q1]  "<mosfet_voltage_Q1>"
  Bus Selector1/1 -> [mosfet_dab_plosses_dab_Q2]  "<mosfet_ploss_Q2>"
  m/1 -> Bus Selector/1, Bus Selector1/1, [inverter_1_dab_mosfet_zvs_modA]

== system sst_dab_ttype_inv/dab_modA/dcdc_with_galvanic_isolation/full-bridge_2/full-bridge_ideal_switch_based/data_measure ==
  m : Inport
  Bus Selector1 : BusSelector  OutputSignals=ideal_switch_current_Q2,ideal_switch_voltage_Q2
  Bus Selector2 : BusSelector  OutputSignals=ideal_switch_current_Q1,ideal_switch_voltage_Q1
  tag scope: idevice_ids_dab_Q5_modA=global, idevice_ids_dab_Q6_modA=global, idevice_uds_dab_Q5_modA=global, idevice_uds_dab_Q6_modA=global
  wires:
  Bus Selector1/1 -> [idevice_ids_dab_Q6_modA]  "<ideal_switch_current_Q2>"
  Bus Selector1/2 -> [idevice_uds_dab_Q6_modA]  "<ideal_switch_voltage_Q2>"
  m/1 -> Bus Selector2/1, Bus Selector1/1
  Bus Selector2/1 -> [idevice_ids_dab_Q5_modA]  "<ideal_switch_current_Q1>"
  Bus Selector2/2 -> [idevice_uds_dab_Q5_modA]  "<ideal_switch_voltage_Q1>"

== system sst_dab_ttype_inv/dab_modA/dcdc_with_galvanic_isolation/full-bridge_2/full-bridge_mosfet_based_with_thermal_model/data_measure ==
  m : Inport
  Bus Selector : BusSelector  OutputSignals=mosfet_ploss_Q1,mosfet_voltage_Q1,mosfet_current_Q1,mosfet_JH_temp_Q1,mosfet_HA_temp_Q1
  Bus Selector1 : BusSelector  OutputSignals=mosfet_ploss_Q2,mosfet_voltage_Q2,mosfet_current_Q2,mosfet_JH_temp_Q2,mosfet_HA_temp_Q2
  tag scope: inverter_2_dab_mosfet_modA=global, mosfet_HA_temp_dab_Q5=global, mosfet_HA_temp_dab_Q6=global, mosfet_JH_temp_dab_Q5=global, mosfet_JH_temp_dab_Q6=global, mosfet_ids_dab_Q5=global, mosfet_ids_dab_Q6=global, mosfet_plosses_dab_Q5=global, mosfet_plosses_dab_Q6=global, mosfet_uds_dab_Q5=global, mosfet_uds_dab_Q6=global
  wires:
  Bus Selector/1 -> [mosfet_plosses_dab_Q5]  "<mosfet_ploss_Q1>"
  Bus Selector1/3 -> [mosfet_ids_dab_Q6]  "<mosfet_current_Q2>"
  Bus Selector1/2 -> [mosfet_uds_dab_Q6]  "<mosfet_voltage_Q2>"
  Bus Selector1/5 -> [mosfet_HA_temp_dab_Q6]  "<mosfet_HA_temp_Q2>"
  Bus Selector/4 -> [mosfet_JH_temp_dab_Q5]  "<mosfet_JH_temp_Q1>"
  Bus Selector/5 -> [mosfet_HA_temp_dab_Q5]  "<mosfet_HA_temp_Q1>"
  Bus Selector1/4 -> [mosfet_JH_temp_dab_Q6]  "<mosfet_JH_temp_Q2>"
  Bus Selector/3 -> [mosfet_ids_dab_Q5]  "<mosfet_current_Q1>"
  Bus Selector/2 -> [mosfet_uds_dab_Q5]  "<mosfet_voltage_Q1>"
  Bus Selector1/1 -> [mosfet_plosses_dab_Q6]  "<mosfet_ploss_Q2>"
  m/1 -> Bus Selector/1, Bus Selector1/1, [inverter_2_dab_mosfet_modA]

== system sst_dab_ttype_inv/dab_modA/dcdc_with_galvanic_isolation/full-bridge_2/full-bridge_mosfet_based_with_thermal_model_zvs/data_measure ==
  m : Inport
  Bus Selector : BusSelector  OutputSignals=mosfet_ploss_Q1,mosfet_voltage_Q1,mosfet_current_Q1,mosfet_JH_temp_Q1,mosfet_HA_temp_Q1
  Bus Selector1 : BusSelector  OutputSignals=mosfet_ploss_Q2,mosfet_voltage_Q2,mosfet_current_Q2,mosfet_JH_temp_Q2,mosfet_HA_temp_Q2
  tag scope: inverter_2_dab_mosfet_zvs_modA=global, mosfet_dab_HA_temp_dab_Q5=global, mosfet_dab_HA_temp_dab_Q6=global, mosfet_dab_JH_temp_dab_Q5=global, mosfet_dab_JH_temp_dab_Q6=global, mosfet_dab_ids_dab_Q5=global, mosfet_dab_ids_dab_Q6=global, mosfet_dab_plosses_dab_Q5=global, mosfet_dab_plosses_dab_Q6=global, mosfet_dab_uds_dab_Q5=global, mosfet_dab_uds_dab_Q6=global
  wires:
  Bus Selector/1 -> [mosfet_dab_plosses_dab_Q5]  "<mosfet_ploss_Q1>"
  Bus Selector1/3 -> [mosfet_dab_ids_dab_Q6]  "<mosfet_current_Q2>"
  Bus Selector1/2 -> [mosfet_dab_uds_dab_Q6]  "<mosfet_voltage_Q2>"
  Bus Selector1/5 -> [mosfet_dab_HA_temp_dab_Q6]  "<mosfet_HA_temp_Q2>"
  Bus Selector/4 -> [mosfet_dab_JH_temp_dab_Q5]  "<mosfet_JH_temp_Q1>"
  Bus Selector/5 -> [mosfet_dab_HA_temp_dab_Q5]  "<mosfet_HA_temp_Q1>"
  Bus Selector1/4 -> [mosfet_dab_JH_temp_dab_Q6]  "<mosfet_JH_temp_Q2>"
  Bus Selector/3 -> [mosfet_dab_ids_dab_Q5]  "<mosfet_current_Q1>"
  Bus Selector/2 -> [mosfet_dab_uds_dab_Q5]  "<mosfet_voltage_Q1>"
  Bus Selector1/1 -> [mosfet_dab_plosses_dab_Q6]  "<mosfet_ploss_Q2>"
  m/1 -> Bus Selector/1, Bus Selector1/1, [inverter_2_dab_mosfet_zvs_modA]

== system sst_dab_ttype_inv/dab_modB/dcdc_with_galvanic_isolation/full-bridge_1/full-bridge_ideal_switch_based/data_measure ==
  m : Inport
  Bus Selector1 : BusSelector  OutputSignals=ideal_switch_current_Q2,ideal_switch_voltage_Q2
  Bus Selector2 : BusSelector  OutputSignals=ideal_switch_current_Q1,ideal_switch_voltage_Q1
  tag scope: idevice_ids_dab_Q1_modB=global, idevice_ids_dab_Q2_modB=global, idevice_uds_dab_Q1_modB=global, idevice_uds_dab_Q2_modB=global
  wires:
  Bus Selector2/2 -> [idevice_uds_dab_Q1_modB]  "<ideal_switch_voltage_Q1>"
  Bus Selector2/1 -> [idevice_ids_dab_Q1_modB]  "<ideal_switch_current_Q1>"
  m/1 -> Bus Selector1/1, Bus Selector2/1
  Bus Selector1/2 -> [idevice_uds_dab_Q2_modB]  "<ideal_switch_voltage_Q2>"
  Bus Selector1/1 -> [idevice_ids_dab_Q2_modB]  "<ideal_switch_current_Q2>"

== system sst_dab_ttype_inv/dab_modB/dcdc_with_galvanic_isolation/full-bridge_1/full-bridge_mosfet_based_with_thermal_model/data_measure ==
  m : Inport
  Bus Selector : BusSelector  OutputSignals=mosfet_ploss_Q1,mosfet_voltage_Q1,mosfet_current_Q1,mosfet_JH_temp_Q1,mosfet_HA_temp_Q1
  Bus Selector1 : BusSelector  OutputSignals=mosfet_ploss_Q2,mosfet_voltage_Q2,mosfet_current_Q2,mosfet_JH_temp_Q2,mosfet_HA_temp_Q2
  tag scope: inverter_1_dab_mosfet_modA=global, mosfet_HA_temp_dab_Q1=global, mosfet_HA_temp_dab_Q2=global, mosfet_JH_temp_dab_Q1=global, mosfet_JH_temp_dab_Q2=global, mosfet_ids_dab_Q1=global, mosfet_ids_dab_Q2=global, mosfet_plosses_dab_Q1=global, mosfet_plosses_dab_Q2=global, mosfet_uds_dab_Q1=global, mosfet_uds_dab_Q2=global
  wires:
  m/1 -> [inverter_1_dab_mosfet_modA], Bus Selector1/1, Bus Selector/1
  Bus Selector1/1 -> [mosfet_plosses_dab_Q2]  "<mosfet_ploss_Q2>"
  Bus Selector/2 -> [mosfet_uds_dab_Q1]  "<mosfet_voltage_Q1>"
  Bus Selector/3 -> [mosfet_ids_dab_Q1]  "<mosfet_current_Q1>"
  Bus Selector1/4 -> [mosfet_JH_temp_dab_Q2]  "<mosfet_JH_temp_Q2>"
  Bus Selector/5 -> [mosfet_HA_temp_dab_Q1]  "<mosfet_HA_temp_Q1>"
  Bus Selector/4 -> [mosfet_JH_temp_dab_Q1]  "<mosfet_JH_temp_Q1>"
  Bus Selector1/5 -> [mosfet_HA_temp_dab_Q2]  "<mosfet_HA_temp_Q2>"
  Bus Selector1/2 -> [mosfet_uds_dab_Q2]  "<mosfet_voltage_Q2>"
  Bus Selector1/3 -> [mosfet_ids_dab_Q2]  "<mosfet_current_Q2>"
  Bus Selector/1 -> [mosfet_plosses_dab_Q1]  "<mosfet_ploss_Q1>"

== system sst_dab_ttype_inv/dab_modB/dcdc_with_galvanic_isolation/full-bridge_1/full-bridge_mosfet_based_with_thermal_model_zvs/data_measure ==
  m : Inport
  tag scope: inverter_1_dab_mosfet_zvs_modB=global
  wires:
  m/1 -> [inverter_1_dab_mosfet_zvs_modB]

== system sst_dab_ttype_inv/dab_modB/dcdc_with_galvanic_isolation/full-bridge_2/full-bridge_ideal_switch_based/data_measure ==
  m : Inport
  Bus Selector1 : BusSelector  OutputSignals=ideal_switch_current_Q2,ideal_switch_voltage_Q2
  Bus Selector2 : BusSelector  OutputSignals=ideal_switch_current_Q1,ideal_switch_voltage_Q1
  tag scope: idevice_ids_dab_Q5_modB=global, idevice_ids_dab_Q6_modB=global, idevice_uds_dab_Q5_modB=global, idevice_uds_dab_Q6_modB=global
  wires:
  Bus Selector2/2 -> [idevice_uds_dab_Q5_modB]  "<ideal_switch_voltage_Q1>"
  Bus Selector2/1 -> [idevice_ids_dab_Q5_modB]  "<ideal_switch_current_Q1>"
  m/1 -> Bus Selector1/1, Bus Selector2/1
  Bus Selector1/2 -> [idevice_uds_dab_Q6_modB]  "<ideal_switch_voltage_Q2>"
  Bus Selector1/1 -> [idevice_ids_dab_Q6_modB]  "<ideal_switch_current_Q2>"

== system sst_dab_ttype_inv/dab_modB/dcdc_with_galvanic_isolation/full-bridge_2/full-bridge_mosfet_based_with_thermal_model/data_measure ==
  m : Inport
  tag scope: inverter_2_dab_mosfet_modB=global
  wires:
  m/1 -> [inverter_2_dab_mosfet_modB]

== system sst_dab_ttype_inv/dab_modB/dcdc_with_galvanic_isolation/full-bridge_2/full-bridge_mosfet_based_with_thermal_model_zvs/data_measure ==
  m : Inport
  tag scope: inverter_2_dab_mosfet_zvs_modB=global
  wires:
  m/1 -> [inverter_2_dab_mosfet_zvs_modB]

== system sst_dab_ttype_inv/single_phase_inverter_modA/single phase inverter control/single_phase_inverter_ctrl/single_phase_current_control/current_reference_generation ==
  mag_ref : Inport
  phase : Inport  Port=2
  Bus Creator : BusCreator  Inputs=2
  Product : Product
  Product1 : Product
  Sin : Trigonometry  Operator=cos
  Sin1 : Trigonometry
  is_ref : Outport
  id_ref : Outport  Port=2
  wires:
  Sin/1 -> Product/2
  phase/1 -> Sin1/1, Sin/1
  mag_ref/1 -> id_ref/1, Product1/1, Product/1
  Sin1/1 -> Product1/2
  Product/1 -> Bus Creator/1  "is_ref_alpha"
  Product1/1 -> Bus Creator/2  "is_ref_beta"
  Bus Creator/1 -> is_ref/1

== system sst_dab_ttype_inv/single_phase_inverter_modA/single phase inverter control/single_phase_inverter_ctrl/single_phase_current_control/dqpi_current_controller ==
  id_ref : Inport
  Bus Creator : BusCreator  Inputs=3
  Bus Creator1 : BusCreator  Inputs=3
  alpha_beta currents : Scope  NumInputPorts=3
      settings: ActiveDisplayYMinimum=-3.07452392578125  ActiveDisplayYMaximum=2.19708251953125  DataLoggingVariableName=ScopeData2
  alphabeta2dq : Subsystem
  dq2alphabeta : Subsystem
  dq_vector_pi : Subsystem
  dq_vector_pi_tracking : Scope  NumInputPorts=2
      settings: ActiveDisplayYMinimum=-5.8450231123834442  ActiveDisplayYMaximum=20.947282871449747  DataLoggingVariableName=ScopeData8
  i2alphabeta : Subsystem
  u_out : Outport
  tag scope: i_alpha=scoped, i_beta=scoped, id=scoped, id_ref=scoped, iq=scoped, ud_ctrl=scoped, uq_ctrl=scoped
  wires:
  dq2alphabeta/1(alpha) -> u_out/1
  id_ref/1 -> dq_vector_pi/1(id_ref), Bus Creator/1, [id_ref]
  alphabeta2dq/1("d ") -> Bus Creator/2, [id], dq_vector_pi/2(id)  "id"
  alphabeta2dq/2("q ") -> dq_vector_pi/3(iq), Bus Creator1/2, [iq]  "iq"
  [iq_ref] -> dq_vector_pi/4(iq_ref)
  Bus Creator1/1 -> dq_vector_pi_tracking/2
  Bus Creator/1 -> dq_vector_pi_tracking/1
  [ud_ctrl] -> Bus Creator/3
  [uq_ctrl] -> Bus Creator1/3
  [iq_ref] -> Bus Creator1/1
  [afe_current_output_pu] -> alpha_beta currents/1, i2alphabeta/1(i_alpha)  "i_load"
  i2alphabeta/1(i_alpha_out) -> alpha_beta currents/2, [i_alpha], alphabeta2dq/1(alpha)  "i_alpha"
  i2alphabeta/2(i_beta_out) -> [i_beta], alpha_beta currents/3, alphabeta2dq/2(beta)  "i_beta"
  dq_vector_pi/1(ud_ctrl) -> [ud_ctrl], dq2alphabeta/1(d)
  dq_vector_pi/2(uq_ctrl) -> [uq_ctrl], dq2alphabeta/2(q)

== system sst_dab_ttype_inv/single_phase_inverter_modA/single phase inverter control/single_phase_inverter_ctrl/single_phase_pll/double_integrator_observer ==
  theta : Inport
  Gain : Gain  Gain=afe_ctrl.di_obs.Ldso  Multiplication=Matrix(K*u)
  Gain1 : Gain  Gain=afe_ctrl.di_obs.Adso  Multiplication=Matrix(K*u)
  Gain2 : Gain  Gain=afe_ctrl.di_obs.Cso  Multiplication=Matrix(K*u)
  Selector : Selector  InputPortWidth=2  IndexOptions=Index vector (dialog)  Indices=2  OutputSizes=1
  Sum : Sum  Inputs=-+|
  Sum1 : Sum  Inputs=|++
  Unit Delay : UnitDelay  SampleTime=-1
  bounder1 : MATLAB Function  TreatAsAtomicUnit=on
  bounder2 : MATLAB Function  TreatAsAtomicUnit=on
  kp3 : Gain  Gain=1/grid_emu.omega_grid_nom  SaturateOnIntegerOverflow=on  OutDataTypeStr=Inherit: Same as input  ParamDataTypeStr=Inherit: Same as input
  phase_hat : Outport
  omega_hat : Outport  Port=2
  wires:
  Gain/1 -> Sum1/1
  Gain2/1 -> bounder2/1(u)  "theta_hat"
  Gain1/1 -> Sum1/2
  Sum1/1 -> Unit Delay/1
  Sum/1 -> bounder1/1(u)  "e"
  Unit Delay/1 -> Selector/1, Gain1/1, Gain2/1
  theta/1 -> Sum/2  "theta"
  bounder1/1(y) -> Gain/1  "e_bounded"
  bounder2/1(y) -> phase_hat/1, Sum/1  "theta_hat_bounded"
  Selector/1 -> kp3/1
  kp3/1 -> omega_hat/1

== system sst_dab_ttype_inv/single_phase_inverter_modA/single phase inverter control/single_phase_inverter_ctrl/single_phase_pll/pi-ctrl ==
  x : Inport
  xref : Inport  Port=2
  1/Ti : Gain  Gain=kp  SaturateOnIntegerOverflow=on  OutDataTypeStr=Inherit: Same as input  ParamDataTypeStr=Inherit: Same as input
  Saturation : Saturate  UpperLimit=sat_pos  LowerLimit=sat_neg
  Sum1 : Sum  Inputs=+++  SaturateOnIntegerOverflow=on
  Sum2 : Sum  Inputs=-+  SaturateOnIntegerOverflow=on
  Sum3 : Sum  Inputs=-+  SaturateOnIntegerOverflow=on
  Unit Delay4 : UnitDelay  SampleTime=-1
  kp : Gain  Gain=ki*ts  SaturateOnIntegerOverflow=on  OutDataTypeStr=Inherit: Same as input  ParamDataTypeStr=Inherit: Same as input
  u : Outport
  wires:
  Saturation/1 -> Sum3/2, u/1
  Unit Delay4/1 -> Sum1/3
  Sum1/1 -> Saturation/1
  Sum3/1 -> Unit Delay4/1
  1/Ti/1 -> Sum3/1, Sum1/1
  Sum2/1 -> 1/Ti/1, kp/1
  kp/1 -> Sum1/2
  x/1 -> Sum2/1
  xref/1 -> Sum2/2

== system sst_dab_ttype_inv/single_phase_inverter_modB/single phase inverter control/single_phase_inverter_ctrl/single_phase_current_control/current_reference_generation ==
  mag_ref : Inport
  phase : Inport  Port=2
  Bus Creator : BusCreator  Inputs=2
  Product : Product
  Product1 : Product
  Sin : Trigonometry  Operator=cos
  Sin1 : Trigonometry
  is_ref : Outport
  id_ref : Outport  Port=2
  wires:
  Bus Creator/1 -> is_ref/1
  Product1/1 -> Bus Creator/2  "is_ref_beta"
  Product/1 -> Bus Creator/1  "is_ref_alpha"
  Sin1/1 -> Product1/2
  mag_ref/1 -> Product/1, Product1/1, id_ref/1
  phase/1 -> Sin/1, Sin1/1
  Sin/1 -> Product/2
